simulink model "Antialias0"  (R2025b)
settings: Solver=VariableStepAuto  StartTime=0.0  StopTime=1  RelTol=1e-3
InitFcn:
  | % -------------------------------------------------------------------------
  | %  [1.6] Filtro Anti-aliasing Analógico
  | % -------------------------------------------------------------------------
  | R1_aa = 150e3;    % (Ohm)
  | R2_aa = 12e3;     % (Ohm)
  | R3_aa = 30e3;     % (Ohm)
  | C1_aa = 47e-9;    % (F)
  | C2_aa = 3.3e-9;  % (F)
  | % -------------------------------------------------------------------------
  | %  [1.11] Operacional
  | % -------------------------------------------------------------------------
  | Vmin = 0;
  | Vmax = 5;
  | SR   = 4.3e6;
  | Rin  = 35e6;
  | Rout = 20;
  | Gain = 10^(90/20);
  | BW   = 8e6/Gain;
libraries: fl_lib x11, nesl_utility x4, ee_lib x1
settings Model: Creator=elias  LastModifiedBy=elias
settings DataIOCC: SaveOutput=off  SaveTime=off

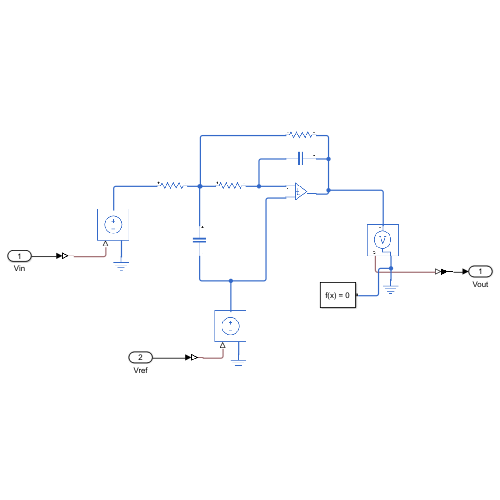
[thumbnail: Simulink's stored preview of the top-level diagram]
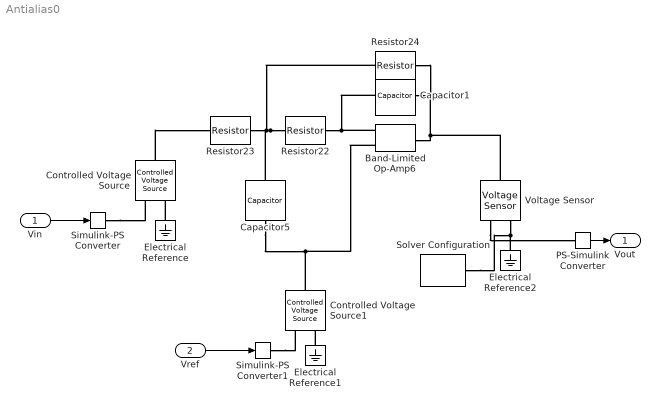
== system Antialias0 ==
  Vin : Inport  OutDataTypeStr=double  PortDimensions=1  SampleTime=0
  Vref : Inport  Port=2  OutDataTypeStr=double  PortDimensions=1
  Band-Limited Op-Amp6 : ee_lib/Integrated Circuits/Band-Limited Op-Amp  A=Gain  Rin=Rin Ohm  Rout=Rout Ohm  Vmin=Vmin V  Vmax=Vmax V  Vdotmax=SR V/s  f=BW Hz  V0=2.5 V
  Capacitor1 : fl_lib/Electrical/Electrical Elements/Capacitor  c=C2_aa F  r=0 Ohm  g=0 1/Ohm  i_specify=off  i_priority=None  i=0 A  i_nominal_specify=off  i_nominal_value=1  i_nominal_unit=A  v_specify=off  v_priority=None  v=0 V  v_nominal_specify=off  v_nominal_value=1  v_nominal_unit=V  vc_specify=off  vc_priority=High  vc=0 V  vc_nominal_specify=off  vc_nominal_value=1  vc_nominal_unit=V
  Capacitor5 : fl_lib/Electrical/Electrical Elements/Capacitor  c=C1_aa F  r=0 Ohm  g=0 1/Ohm  i_specify=off  i_priority=None  i=0 A  i_nominal_specify=off  i_nominal_value=1  i_nominal_unit=A  v_specify=off  v_priority=None  v=0 V  v_nominal_specify=off  v_nominal_value=1  v_nominal_unit=V  vc_specify=off  vc_priority=High  vc=0 V  vc_nominal_specify=off  vc_nominal_value=1  vc_nominal_unit=V
  Controlled Voltage Source : fl_lib/Electrical/Electrical Sources/Controlled Voltage Source
  Controlled Voltage Source1 : fl_lib/Electrical/Electrical Sources/Controlled Voltage Source
  Electrical Reference : fl_lib/Electrical/Electrical Elements/Electrical Reference
  Electrical Reference1 : fl_lib/Electrical/Electrical Elements/Electrical Reference
  Electrical Reference2 : fl_lib/Electrical/Electrical Elements/Electrical Reference
  PS-Simulink Converter : nesl_utility/PS-Simulink Converter  PhysicalDomain=network_engine_domain  SubClassName=ps_output  LeftPortType=input  RightPortType=output  PseudoPeriodic=off  Frequencies=[]  VectorFormat=inherit  Unit=inherit  AffineConversion=off
  Resistor22 : fl_lib/Electrical/Electrical Elements/Resistor  R=R2_aa Ohm  i_specify=off  i_priority=None  i=0 A  i_nominal_specify=off  i_nominal_value=1  i_nominal_unit=A  v_specify=off  v_priority=None  v=0 V  v_nominal_specify=off  v_nominal_value=1  v_nominal_unit=V
  Resistor23 : fl_lib/Electrical/Electrical Elements/Resistor  R=R3_aa Ohm  i_specify=off  i_priority=None  i=0 A  i_nominal_specify=off  i_nominal_value=1  i_nominal_unit=A  v_specify=off  v_priority=None  v=0 V  v_nominal_specify=off  v_nominal_value=1  v_nominal_unit=V
  Resistor24 : fl_lib/Electrical/Electrical Elements/Resistor  R=R1_aa Ohm  i_specify=off  i_priority=None  i=0 A  i_nominal_specify=off  i_nominal_value=1  i_nominal_unit=A  v_specify=off  v_priority=None  v=0 V  v_nominal_specify=off  v_nominal_value=1  v_nominal_unit=V
  Simulink-PS Converter : nesl_utility/Simulink-PS Converter  PhysicalDomain=network_engine_domain  SubClassName=ps_input  LeftPortType=input  RightPortType=output  PseudoPeriodic=off  Frequencies=[]  NoiseDistribution=none  NoiseParameters=[]  Unit=1  AffineConversion=off  FilteringAndDerivatives=provide  SimscapeFilterOrder=1  InputFilterTimeConstant=0.001  UdotUserProvided=0
  Simulink-PS Converter1 : nesl_utility/Simulink-PS Converter  PhysicalDomain=network_engine_domain  SubClassName=ps_input  LeftPortType=input  RightPortType=output  PseudoPeriodic=off  Frequencies=[]  NoiseDistribution=none  NoiseParameters=[]  Unit=1  AffineConversion=off  FilteringAndDerivatives=provide  SimscapeFilterOrder=1  InputFilterTimeConstant=0.001  UdotUserProvided=0
  Solver Configuration : nesl_utility/Solver Configuration  PhysicalDomain=network_engine_domain  SubClassName=solver  LeftPortType=input  RightPortType=generic  Tones=[]  Harmonics=[]  SimulateNoise=off  Profile=off  UseLocalSampling=off  EnableSwitchedLinearOptims=on  FrequencyDomain=off  UseCCode=off  RelTol=0.001  AbsTol=0.001  MinStep=1e-09  ToWorkspace=off  RevertToSquareIcSolve=off  NumHomotopyIterations=100  PhasorMode=off  PhasorModeNumHarmonics=1  ConsistencySolver=NEWTON_XTOL_AFTER_FTOL  IndexReductionMethod=DerivativeReplacement  DoDC=off  ResidualTolerance=1e-09  ConsistencyTolSource=GLOBAL  ConsistencyAbsTol=0.001  ConsistencyRelTol=0.001  ConsistencyTolFactor=0.001  UseLocalSolver=off  LocalSolverChoice=NE_BACKWARD_EULER_ADVANCER  ResolveIndetEquations=on  FunctionEvalNumThread=1  LocalSolverSampleTime=0.001  DoFixedCost=off  MaxNonlinIter=3  MaxModeIter=2  ComputeImpulses=off  ImpulseIterations=2  LinearAlgebra=auto  LinearAlgebraNumThread=0  EquationFormulation=NE_TIME_EF  DelaysMemoryBudget=1024  AutomaticFiltering=on  FilteringTimeConstant=0.001  PartitionStorageMethod=AS_NEEDED  PartitionMemoryBudget=1024  PartitionMethod=ROBUST  MultibodyUseLocalSolver=off  MultibodyLocalSolverChoice=ODE1  MultibodyLocalSolverSampleTime=0.001
  Voltage Sensor : fl_lib/Electrical/Electrical Sensors/Voltage Sensor
  Vout : Outport  OutDataTypeStr=double  PortDimensions=1  SampleTime=0
  wires:
  Vin/1 -> Simulink-PS Converter/1
  Vref/1 -> Simulink-PS Converter1/1
  PS-Simulink Converter/1 -> Vout/1
  connections:
  Resistor22/LConn1 -- Resistor23/RConn1 -- Capacitor5/LConn1 -- Resistor24/LConn1
  Voltage Sensor/LConn1 -- Capacitor1/RConn1 -- Resistor24/RConn1 -- Band-Limited Op-Amp6/RConn1
  Controlled Voltage Source1/LConn1 -- Band-Limited Op-Amp6/LConn1 -- Capacitor5/RConn1
  Band-Limited Op-Amp6/LConn2 -- Resistor22/RConn1 -- Capacitor1/LConn1
  Solver Configuration/RConn1 -- Voltage Sensor/RConn2 -- Electrical Reference2/LConn1
  Controlled Voltage Source/LConn1 -- Resistor23/LConn1
  Electrical Reference/LConn1 -- Controlled Voltage Source/RConn2
  Electrical Reference1/LConn1 -- Controlled Voltage Source1/RConn2
  Simulink-PS Converter/RConn1 -- Controlled Voltage Source/RConn1
  Simulink-PS Converter1/RConn1 -- Controlled Voltage Source1/RConn1
  Voltage Sensor/RConn1 -- PS-Simulink Converter/LConn1
